simulink model "discretoSIMULINK_PD"  (Simulink 7.4)
settings: Solver=ode3  StartTime=0.0  StopTime=20  FixedStep=Ta  RelTol=1e-3
values from neighbouring files (symbols this model uses):
  amplitude = 50    [discreto.m]
  denp = [1 a2 a1 a0]    [discreto.m]
  Kd_PD = K_PD    [discreto.m]
  Ki_PD = 0    [discreto.m]
  Kp_PD = (1/Zero_PD-1)*K_PD/Ta    [discreto.m]
  nump = [0 b2 b1 b0]    [discreto.m]
  ruido_media = 0.011877972928933    (= 0.0118779729289)    [discreto.m]
  ruido_variancia = 0.1    [discreto.m]
  saturacao_max = 5    [discreto.m]
  saturacao_min = -5    [discreto.m]
  Ta = 1/1000    (= 0.001)    [continuo.m]    (also in discreto.m = 0.01)
settings Model: Creator=Fabiano  LastModifiedBy=Fabiano
settings DataIOCC: SignalLoggingName=sigsOut
settings DebuggingCC: SaveWithParameterizedLinksMsg=none  SignalResolutionControl=TryResolveAllWithWarning  SolverPrmCheckMsg=none  MultiTaskDSMMsg=warning  MultiTaskCondExecSysMsg=none  StrictBusMsg=None
settings HardwareCC: TargetUnknown=on
settings RTWCC: IncludeERTFirstTime=on

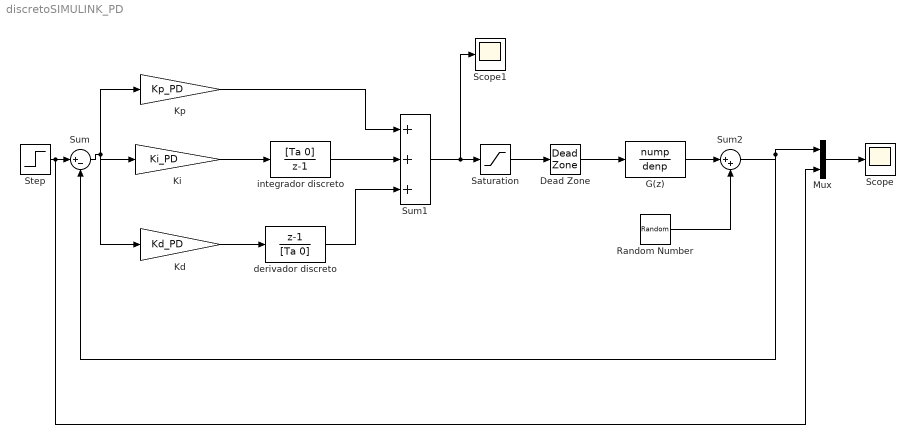
== system discretoSIMULINK_PD ==
  Dead Zone : DeadZone  LowerValue=banda_morta_ini  UpperValue=banda_morta_fim  SaturateOnIntegerOverflow=on
  G(z) : DiscreteTransferFcn  Numerator=nump  Denominator=denp  SampleTime=Ta
  Kd : Gain  Gain=Kd_PD  ParameterDataType=sfix(16)  ParameterScaling=2^0  OutDataType=sfix(16)  OutScaling=2^0  SaturateOnIntegerOverflow=on  OutDataTypeStr=Inherit: Same as input  ParamDataTypeStr=Inherit: Same as input
  Ki : Gain  Gain=Ki_PD  ParameterDataType=sfix(16)  ParameterScaling=2^0  OutDataType=sfix(16)  OutScaling=2^0  SaturateOnIntegerOverflow=on  OutDataTypeStr=Inherit: Same as input  ParamDataTypeStr=Inherit: Same as input
  Kp : Gain  Gain=Kp_PD  ParameterDataType=sfix(16)  ParameterScaling=2^0  OutDataType=sfix(16)  OutScaling=2^0  SaturateOnIntegerOverflow=on  OutDataTypeStr=Inherit: Same as input  ParamDataTypeStr=Inherit: Same as input
  Mux : Mux  Inputs=2
  Random Number : RandomNumber  Mean=ruido_media  Variance=ruido_variancia  SampleTime=0
  Saturation : Saturate  UpperLimit=saturacao_max  LowerLimit=saturacao_min
  Scope : Scope
      settings: TimeRange=10  SaveName=sinais  DataFormat=Array
  Scope1 : Scope
      settings: TimeRange=10  YMin=-1
  Step : Step  Time=0  After=amplitude  SampleTime=0
  Sum : Sum  Inputs=|+-  OutDataType=sfix(16)  OutScaling=2^0  SaturateOnIntegerOverflow=on
  Sum1 : Sum  Inputs=+++  OutDataType=sfix(16)  OutScaling=2^0  SaturateOnIntegerOverflow=on
  Sum2 : Sum  Inputs=|++  OutDataType=sfix(16)  OutScaling=2^0  SaturateOnIntegerOverflow=on
  derivador discreto : DiscreteTransferFcn  Numerator=[1 -1]  Denominator=[Ta 0]  SampleTime=Ta
  integrador discreto : DiscreteTransferFcn  Numerator=[Ta 0]  Denominator="[1  -1]"  SampleTime=Ta
  wires:
  Saturation/1 -> Dead Zone/1
  Step/1 -> Sum/1, Mux/2
  Kp/1 -> Sum1/1
  integrador discreto/1 -> Sum1/2
  Ki/1 -> integrador discreto/1
  Kd/1 -> derivador discreto/1
  Sum/1 -> Kp/1, Kd/1, Ki/1
  Sum1/1 -> Saturation/1, Scope1/1
  Mux/1 -> Scope/1
  G(z)/1 -> Sum2/1
  Random Number/1 -> Sum2/2
  Sum2/1 -> Mux/1, Sum/2
  derivador discreto/1 -> Sum1/3
  Dead Zone/1 -> G(z)/1
